simulink model "sbw_actuator_2023a"  (R2022b)
settings: Solver=ode5  StartTime=0.0  StopTime=100  FixedStep=0.0001  RelTol=1e-3
InitFcn:
  | %% 转向执行总成参数
  | % 电机输出轴
  | I_sam = 0.02;                 % kg·m^2
  | B_sam = 0.002 * 180/pi;                 % N·m·s/rad
  | K_fsam = 0.2;                  % N·m
  | 
  | % 齿条
  | M_sr = 32.47;                     % kg
  | B_sr = 5500;                     % N·s/m
  | K_fsr =300;                     % N
  | 
  | % 结构参数
  | k_bm = 17600;                     % N·m/rad
  | i_bs =  111.7011;         % rad/m
libraries: Solver_SF x1
settings Model: Creator=23649  LastModifiedBy=23649
settings OptimizationCC: ReuseModelBlockBuffer=on
settings RTWCC: GPUComputeCapability=5.0
settings ConfigComp: CovBoundaryAbsTol=1.0e-5

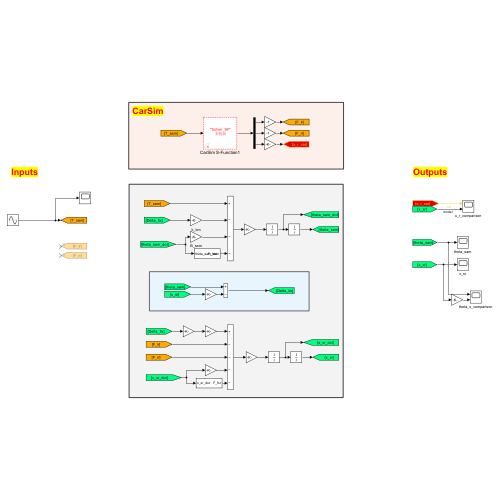
[thumbnail: Simulink's stored preview of the top-level diagram]
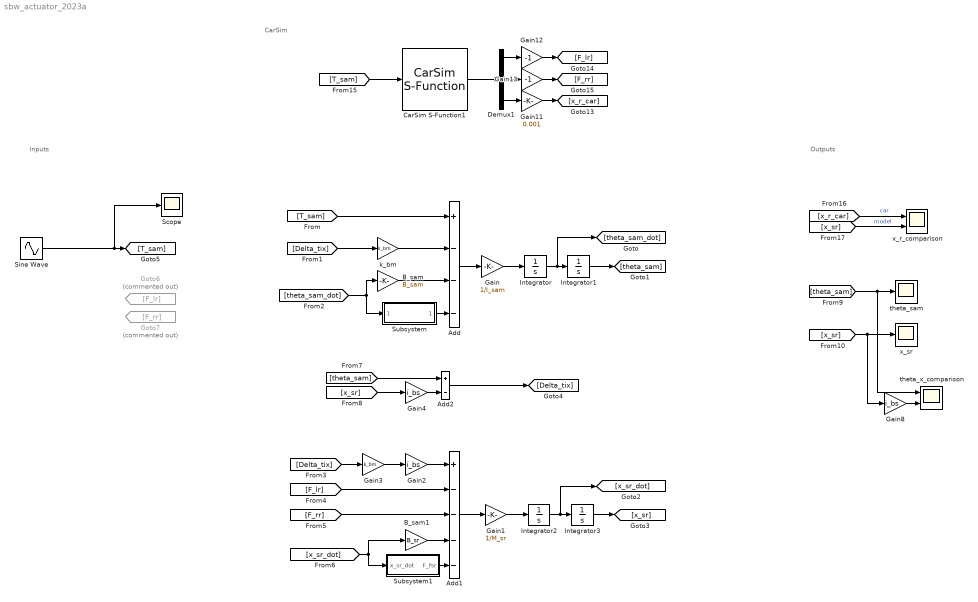
== system sbw_actuator_2023a ==
  note: CarSim
  note: Inputs
  note: Outputs
  Add : Sum  Inputs=+---
  Add1 : Sum  Inputs=+----
  Add2 : Sum  Inputs=+-
  B_sam : Gain  Gain=B_sam
  B_sam1 : Gain  Gain=B_sr
  CarSim S-Function1 : Solver_SF/CarSim S-Function  Priority=1  SIMFILE=simfile.sim  Run_RTs=off  vs_state_ind=Run  StopMode_ind=Vehicle Model
  Demux1 : Demux  Outputs=3
  Gain : Gain  Gain=1/I_sam
  Gain1 : Gain  Gain=1/M_sr
  Gain11 : Gain  Gain=0.001
  Gain12 : Gain  Gain=-1
  Gain13 : Gain  Gain=-1
  Gain2 : Gain  Gain=i_bs
  Gain3 : Gain  Gain=k_bm
  Gain4 : Gain  Gain=i_bs
  Gain8 : Gain  Gain=i_bs
  Goto6 : Goto  Commented=on  GotoTag=F_lr
  Goto7 : Goto  Commented=on  GotoTag=F_rr
  Integrator{,1..3} (4 alike) : Integrator
  Scope : Scope
  Sine Wave : Sin  Amplitude=10  SampleTime=0
  Subsystem : Subsystem
  Subsystem1 : Subsystem
  k_bm : Gain  Gain=k_bm
  theta_sam : Scope
  theta_x_comparison : Scope  NumInputPorts=2
  x_r_comparison : Scope  NumInputPorts=2
  x_sr : Scope
  wires:
  Add/1 -> Gain/1
  Gain/1 -> Integrator/1
  [T_sam] -> Add/1
  k_bm/1 -> Add/2
  [Delta_tix] -> k_bm/1
  B_sam/1 -> Add/3
  [theta_sam_dot] -> B_sam/1, Subsystem/1(theta_sam_dot)
  Subsystem/1(F_fsam) -> Add/4
  Integrator/1 -> Integrator1/1, [theta_sam_dot]
  Integrator1/1 -> [theta_sam]
  Integrator3/1 -> [x_sr]
  Integrator2/1 -> Integrator3/1, [x_sr_dot]
  Gain1/1 -> Integrator2/1
  Add1/1 -> Gain1/1
  [Delta_tix] -> Gain3/1
  Gain2/1 -> Add1/1
  Gain3/1 -> Gain2/1
  [F_lr] -> Add1/2
  [F_rr] -> Add1/3
  B_sam1/1 -> Add1/4
  [x_sr_dot] -> B_sam1/1, Subsystem1/1(x_sr_dot)
  Subsystem1/1(F_fsr) -> Add1/5
  Add2/1 -> [Delta_tix]
  [x_sr] -> Gain4/1
  [theta_sam] -> Add2/1
  Gain4/1 -> Add2/2
  Sine Wave/1 -> Scope/1, [T_sam]
  [theta_sam] -> theta_sam/1, theta_x_comparison/1
  Gain8/1 -> theta_x_comparison/2
  [x_sr] -> Gain8/1, x_sr/1
  CarSim S-Function1/1 -> Demux1/1
  [T_sam] -> CarSim S-Function1/1
  Demux1/3 -> Gain11/1
  Demux1/2 -> Gain13/1
  Demux1/1 -> Gain12/1
  Gain11/1 -> [x_r_car]
  [x_r_car] -> x_r_comparison/1  "car"
  [x_sr] -> x_r_comparison/2  "model"
  Gain12/1 -> [F_lr]
  Gain13/1 -> [F_rr]

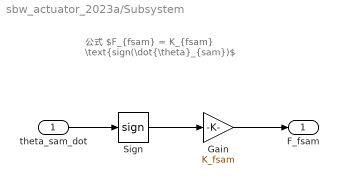
== system sbw_actuator_2023a/Subsystem ==
  note: 公式 $F_{fsam} = K_{fsam} \text{sign(\dot{\theta}_{sam})$
  theta_sam_dot : Inport
  Gain : Gain  Gain=K_fsam
  Sign : Signum
  F_fsam : Outport
  wires:
  theta_sam_dot/1 -> Sign/1
  Gain/1 -> F_fsam/1
  Sign/1 -> Gain/1

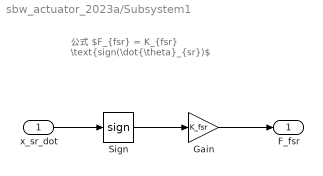
== system sbw_actuator_2023a/Subsystem1 ==
  note: 公式 $F_{fsr} = K_{fsr} \text{sign(\dot{\theta}_{sr})$
  x_sr_dot : Inport
  Gain : Gain  Gain=K_fsr
  Sign : Signum
  F_fsr : Outport
  wires:
  x_sr_dot/1 -> Sign/1
  Gain/1 -> F_fsr/1
  Sign/1 -> Gain/1
